simulink model "FIR_Direct_form_filter"  (R2020b)
settings: Solver=FixedStepAuto  StartTime=0.0  StopTime=10.0  FixedStep=0.2  RelTol=1e-3
settings Model: Creator=ASUS  LastModifiedBy=ASUS
settings DataIOCC: SaveOutput=off  SaveTime=off

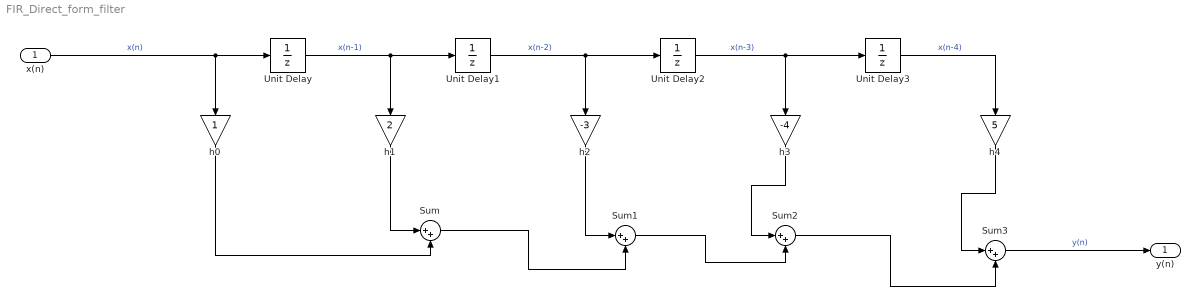
== system FIR_Direct_form_filter ==
  x(n) : Inport  OutDataTypeStr=double  PortDimensions=1  SampleTime=[0.20000000000000001,0]
  Sum{,1..3} (4 alike) : Sum  Inputs=|++
  Unit Delay{,1..3} (4 alike) : UnitDelay  SampleTime=-1  HasFrameUpgradeWarning=on
  h0 : Gain
  h1 : Gain  Gain=2
  h2 : Gain  Gain=-3
  h3 : Gain  Gain=-4
  h4 : Gain  Gain=5
  y(n) : Outport  OutDataTypeStr=double  PortDimensions=1  SampleTime=[0.20000000000000001,0]
  wires:
  Unit Delay1/1 -> Unit Delay2/1, h2/1  "x(n-2)"
  x(n)/1 -> Unit Delay/1, h0/1  "x(n)"
  Sum2/1 -> Sum3/2
  h2/1 -> Sum1/1
  h0/1 -> Sum/2
  Sum1/1 -> Sum2/2
  Unit Delay2/1 -> Unit Delay3/1, h3/1  "x(n-3)"
  Sum/1 -> Sum1/2
  Unit Delay/1 -> Unit Delay1/1, h1/1  "x(n-1)"
  h3/1 -> Sum2/1
  h1/1 -> Sum/1
  Unit Delay3/1 -> h4/1  "x(n-4)"
  h4/1 -> Sum3/1
  Sum3/1 -> y(n)/1  "y(n)"
